simulink model "model_1Sy"  (R2023a)
settings: Solver=VariableStepAuto  StartTime=0.0  StopTime=150  RelTol=1e-3
values from neighbouring files (symbols this model uses):
  b = A(3)    [F1Sy.m]    (also in F1Vexp2V_SexpS.m = A(4); F1Vexp2V_SexpS_ssr.m = abs(b); F1Vexp2V_SexpS_ssr_all.m = input_parameters(5); F1VxSy.m = A(4))
  data = load(input_data)    [F1.m]    (also in F1Sy.m; F1Vexp2V.m; F1Vexp2V_SexpS.m; F1Vexp2V_SexpS_ssr.m)
  R = A(2)    [F1.m]    (also in F1Sy.m; F1Vexp2V.m; F1Vexp2V_SexpS.m; F1Vexp2V_SexpS_ssr_all.m = input_parameters(2))
  y = input_parameters(2)    [F1Vexp2V_SexpS_ssr.m]    (also in F1Vexp2V_SexpS_ssr_all.m = input_parameters(6))
settings Model: Creator=test  LastModifiedBy=test
settings DebuggingCC: AlgebraicLoopMsg=none

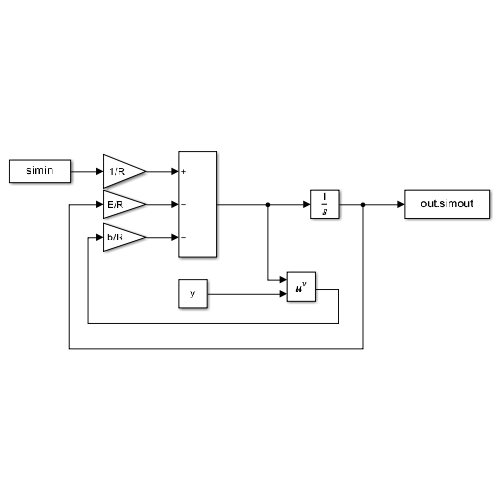
[thumbnail: Simulink's stored preview of the top-level diagram]
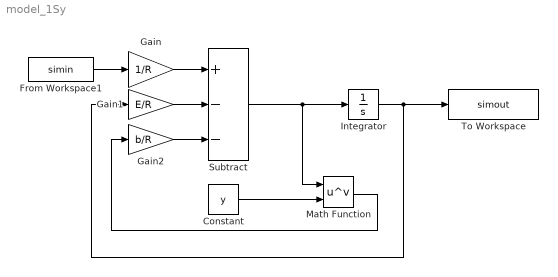
== system model_1Sy ==
  Constant : Constant  Value=y
  From Workspace1 : FromWorkspace  VariableName=simin
  Gain : Gain  Gain=1/R
  Gain1 : Gain  Gain=E/R
  Gain2 : Gain  Gain=b/R
  Integrator : Integrator  InitialCondition=data(1,3)
  Math Function : Math  Operator=pow
  Subtract : Sum  Inputs=+--
  To Workspace : ToWorkspace  VariableName=simout  SaveFormat=Timeseries  SampleTime=0.01
  wires:
  Gain2/1 -> Subtract/3
  Constant/1 -> Math Function/2
  Gain/1 -> Subtract/1
  Subtract/1 -> Math Function/1, Integrator/1
  Integrator/1 -> To Workspace/1, Gain1/1
  From Workspace1/1 -> Gain/1
  Math Function/1 -> Gain2/1
  Gain1/1 -> Subtract/2
